simulink model "ep3_6"  (R2018a)
settings: Solver=VariableStepAuto  StartTime=0.0  StopTime=20  MaxStep=0.1  RelTol=1e-3
settings Model: Creator=zheny  LastModifiedBy=zheny

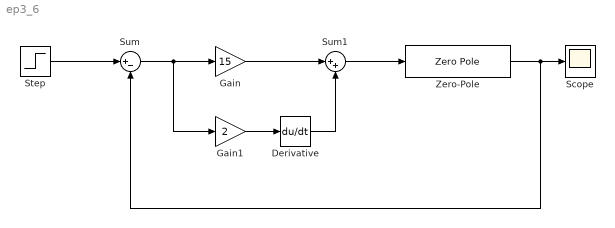
== system ep3_6 ==
  Derivative : Derivative
  Gain : Gain  Gain=15
  Gain1 : Gain  Gain=2
  Scope : Scope
  Step : Step  SampleTime=0
  Sum : Sum  Inputs=|+-
  Sum1 : Sum  Inputs=|++
  Zero-Pole : ZeroPole  Zeros=[]  Poles=[1.1 -1.1]
  wires:
  Step/1 -> Sum/1
  Sum/1 -> Gain1/1, Gain/1
  Gain/1 -> Sum1/1
  Sum1/1 -> Zero-Pole/1
  Zero-Pole/1 -> Sum/2, Scope/1
  Gain1/1 -> Derivative/1
  Derivative/1 -> Sum1/2
